simulink library "RGPBasedRealTimeControl_cl"  (R2020a)
settings: Solver=VariableStepAuto  StartTime=0.0  StopTime=10.0  RelTol=1e-3
libraries: squareWave_ul x1
settings Model: Creator=Ayaz  LastModifiedBy=Ayaz

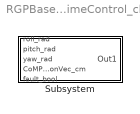
== system RGPBasedRealTimeControl_cl ==
  Subsystem : Subsystem

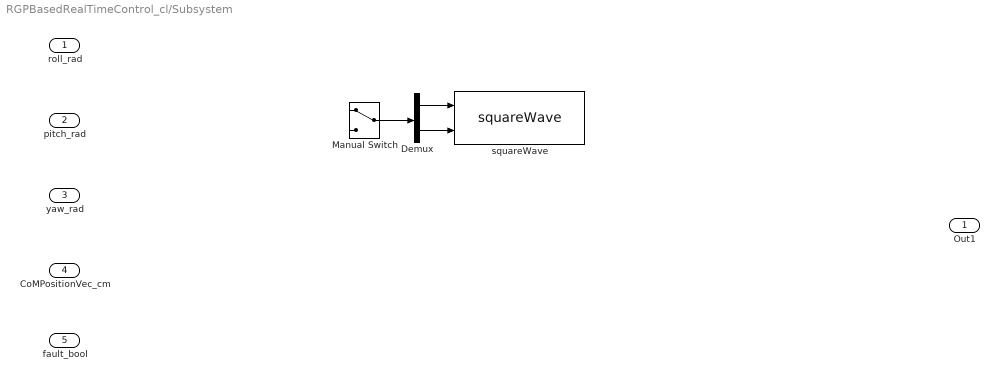
== system RGPBasedRealTimeControl_cl/Subsystem ==
  roll_rad : Inport
  pitch_rad : Inport  Port=2
  yaw_rad : Inport  Port=3
  CoMPositionVec_cm : Inport  Port=4
  fault_bool : Inport  Port=5
  Demux : Demux  Outputs=2
  Manual Switch : ManualSwitch
  squareWave : squareWave_ul/squareWave  startDelay=4
  Out1 : Outport
  wires:
  Demux/1 -> squareWave/1
  Demux/2 -> squareWave/2
  Manual Switch/1 -> Demux/1
